simulink model "motorPosition_PlantModel"  (R2020a)
settings: Solver=VariableStepAuto  StartTime=0.0  StopTime=10.0  RelTol=1e-3
values from neighbouring files (symbols this model uses):
  b = 3.5077E-6    [motor_parameter.sldd]
  J = 3.3384E-6    [motor_parameter.sldd]
  L = 2.75E-6    [motor_parameter.sldd]
  R = 4.0    [motor_parameter.sldd]
undefined symbols (not defined in the file or in its folder): Ke, Kt
settings Model: Creator=INDRAJIT MARATHE  LastModifiedBy=INDRAJIT MARATHE

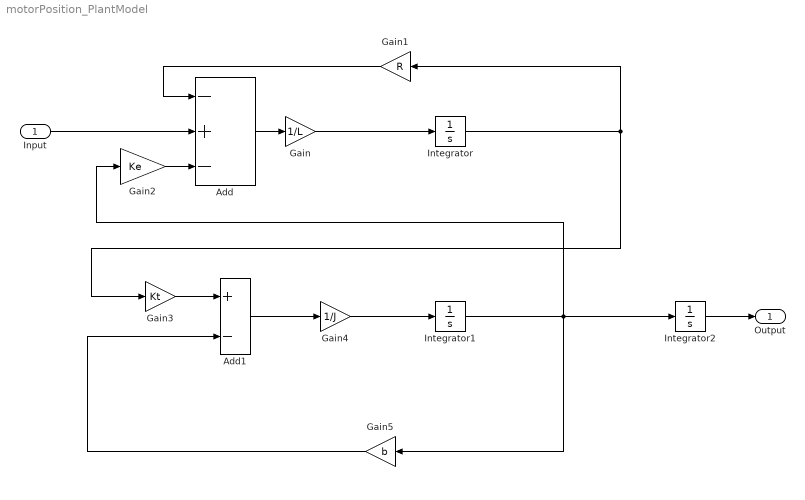
== system motorPosition_PlantModel ==
  Input : Inport
  Add : Sum  Inputs=-+-
  Add1 : Sum  Inputs=+-
  Gain : Gain  Gain=1/L
  Gain1 : Gain  Gain=R
  Gain2 : Gain  Gain=Ke
  Gain3 : Gain  Gain=Kt
  Gain4 : Gain  Gain=1/J
  Gain5 : Gain  Gain=b
  Integrator : Integrator
  Integrator1 : Integrator
  Integrator2 : Integrator
  Output : Outport
  wires:
  Gain3/1 -> Add1/1
  Integrator/1 -> Gain3/1, Gain1/1
  Add1/1 -> Gain4/1
  Gain4/1 -> Integrator1/1
  Integrator1/1 -> Gain2/1, Gain5/1, Integrator2/1
  Integrator2/1 -> Output/1
  Gain/1 -> Integrator/1
  Add/1 -> Gain/1
  Input/1 -> Add/2
  Gain1/1 -> Add/1
  Gain2/1 -> Add/3
  Gain5/1 -> Add1/2
